simulink library "MIL_Test"  (Simulink 6.6)
undefined symbols (not defined in the file or in its folder): getdatatypespecs, slcm, StepSize
libraries: simulink x71, MIL_Test x6
(part 4 of 8)

== system MIL_Test/Validation Function/Feature extraction/Step response characteristics/Step response characteristics extraction/Extract steady state error ==
  Step response : Inport
  Set point : Inport  Port=2
  Subtract : Sum  Inputs=+-  OutScaling=2^-10
  Weighted Moving Average : S-Function  FunctionName=sfix_fir  Parameters=(getdatatypespecs(OutDataType,OutScaling,DblOver,0)),[DoSatur RndMeth-1],DblOver,dolog,mgainval,(getdatatypespecs(GainDataType,GainScaling,DblOver,RadixGroup)),samptime,vinit,OutputDataTypeScalingMode,GainDataTypeScalingMode  mask(Weighted Moving Average){mgainval=ones(1,10), vinit=0.0, samptime=-1, GainDataTypeScalingMode=Inherit via internal rule, GainDataType=sfix( 16 ), MatRadixGroup=Best Precision: Matrix-wise, GainScaling=2^-10, OutputDataTypeScalingMode=Inherit via internal rule, OutDataType=sfix(16), OutScaling=2^-10, LockScale=off, RndMeth=Floor, DoSatur=off}
      mask prompts: mgainval "Weights:"; vinit "Initial condition:"; samptime "Sample time:"; GainDataTypeScalingMode "Gain data type and scaling:"; GainDataType "Parameter data type:     ex. sfix(16),  uint(8), float('single')"; MatRadixGroup "Parameter scaling mode:"; GainScaling "Parameter scaling:    Slope    ex.  2^-9"; OutputDataTypeScalingMode "Output data type and scaling:"; OutDataType "Output data type:     ex.  sfix(16),  uint(8),  float('single')"; OutScaling "Output scaling:    Slope or [Slope Bias]    ex.  2^-9"; LockScale "Lock output scaling so autoscaling tool can't change it"; RndMeth "Round toward:"; DoSatur "Saturate to max or min when overflows occur"
      mask help: Output the weighted moving average of the input.
      mask init:
      | DblOver = 0;
      | dolog = 0;
      | 
      | if MatRadixGroup == 5
      |     RadixGroup = 1; % BEST_PREC_MAT
      | elseif MatRadixGroup == 4
      |     RadixGroup = 2; % BEST_PREC_COL
      | elseif MatRadixGroup == 3
      |     RadixGroup = 3; % BEST_PREC_ROW
      | elseif MatRadixGroup == 2
      |     RadixGroup = 4; % BEST_PREC_ELE
      | else
      |     RadixGroup = 0; % BEST_PREC_OFF
      | end
      mask StyleString: edit,edit,edit,popup(Specify via dialog|Inherit via internal rule),edit,popup(Use Specified Scaling|Best Precision: Element-wise|Best Precision: Row-wise|Best Precision: Column-wise|Best Precision: Matrix-wise),edit,popup(Specify via dialog|Inherit via internal rule|Inherit via back propagation),edit,edit,checkbox,popup(Zero|Nearest|Ceiling|Floor),checkbox
      mask CallbackString: |||fixptdialog(gcbh)|fixptdialog(gcbh)|fixptdialog(gcbh)||fixptdialog(gcbh)|fixptdialog(gcbh)||||
      mask TabNameString: Main,Main,Main,Parameter data types,Parameter data types,Parameter data types,Parameter data types,Signal data types,Signal data types,Signal data types,Signal data types,Signal data types,Signal data types
      mask Display:
      | fprintf(fixpt_fir_mask_data(mgainval,'dispstr'))
      | plot(fixpt_fir_mask_data(mgainval,1),fixpt_fir_mask_data(mgainval,0))
  ss error : Outport
  wires:
  Weighted Moving Average/1 -> ss error/1
  Subtract/1 -> Weighted Moving Average/1
  Set point/1 -> Subtract/2
  Step response/1 -> Subtract/1

== system MIL_Test/Validation Function/Feature extraction/Step response characteristics/Step response characteristics extraction/Step time ==
  Clock : Inport
  Trigger : TriggerPort
  Time : Outport
  wires:
  Clock/1 -> Time/1

== system MIL_Test/Validation Function/Feature extraction/Step response characteristics/Step response reset/Active if signals constant for some specified time ==
  Signal1 : Inport
  Signal 2 : Inport  Port=2
  Logical Operator1 : Logic  AllPortsSameDT=off  OutDataTypeMode=Boolean
  Min Time : Constant
  MinMax : MinMax  Inputs=2
  Relational Operator2 : RelationalOperator  Operator=<=  LogicOutDataTypeMode=Boolean
  Switch : Switch  Criteria=u2 ~= 0
  Time since signal constant : Subsystem  TreatAsAtomicUnit=on  mask(Feature extraction block){RT=0.0001}
      mask prompts: RT "Relative tolerance in %"
      mask help: Detect if the signal value is constant (using the last two signal values) allowing for a user-defined relative deviation
      mask CallbackString:
      | if or( (str2double(get_param(gcb,'RT')) < 0), (str2double(get_param(gcb,'RT')) > 100))
      |     error(['Relative tolerance value (' get_param(gcb,'RT') ') out of range. Please give a value between 0 and 100.']);
      | else
      |     set_param([gcb '/Detect constant/Relative tolerance/Relative Tolerance'],'Value',get_param(gcb,'RT'));
      |     set_param([gcb '/Detect constant'],'RT',get_param(gcb,'RT'));
      | end
  Time since signal constant1 : Subsystem  TreatAsAtomicUnit=on  mask(Feature extraction block){RT=0.0001}
      mask prompts: RT "Relative tolerance in %"
      mask help: Detect if the signal value is constant (using the last two signal values) allowing for a user-defined relative deviation
      mask CallbackString:
      | if or( (str2double(get_param(gcb,'RT')) < 0), (str2double(get_param(gcb,'RT')) > 100))
      |     error(['Relative tolerance value (' get_param(gcb,'RT') ') out of range. Please give a value between 0 and 100.']);
      | else
      |     set_param([gcb '/Detect constant/Relative tolerance/Relative Tolerance'],'Value',get_param(gcb,'RT'));
      |     set_param([gcb '/Detect constant'],'RT',get_param(gcb,'RT'));
      | end
  Zero : Constant  Value=0
  Constant signals : Outport
  wires:
  Zero/1 -> Switch/3
  Logical Operator1/1 -> Switch/2
  MinMax/1 -> Switch/1
  Time since signal constant1/1(Trigger) -> Logical Operator1/2
  Time since signal constant/1(Trigger) -> Logical Operator1/1
  Time since signal constant/2(Feature) -> MinMax/1
  Time since signal constant1/2(Feature) -> MinMax/2
  Switch/1 -> Relational Operator2/2
  Min Time/1 -> Relational Operator2/1
  Relational Operator2/1 -> Constant signals/1
  Signal 2/1 -> Time since signal constant1/1(Signal)
  Signal1/1 -> Time since signal constant/1(Signal)

== system MIL_Test/Validation Function/Feature extraction/Step response characteristics/Step response reset/Step detection ==
  Signal : Inport
  Abs : Abs
  Add : Sum  Inputs=+-  OutScaling=2^-10
  Clock : Clock
      settings: Decimation=10
  Memory : Memory
  Min step size : Constant
  Relational Operator : RelationalOperator  LogicOutDataTypeMode=Boolean
  Switch : Switch  Criteria=u2 > Threshold
  Step : Outport
  wires:
  Switch/1 -> Add/2
  Memory/1 -> Switch/1
  Clock/1 -> Switch/2
  Signal/1 -> Add/1, Switch/3, Memory/1
  Abs/1 -> Relational Operator/1
  Min step size/1 -> Relational Operator/2
  Relational Operator/1 -> Step/1
  Add/1 -> Abs/1

== system MIL_Test/Validation Function/Feature extraction/Step response characteristics/Step response trigger/Active if signals constant for some specified time ==
  Signal1 : Inport
  Signal 2 : Inport  Port=2
  Logical Operator1 : Logic  AllPortsSameDT=off  OutDataTypeMode=Boolean
  Min Time : Constant
  MinMax : MinMax  Inputs=2
  Relational Operator2 : RelationalOperator  Operator=<=  LogicOutDataTypeMode=Boolean
  Switch : Switch  Criteria=u2 ~= 0
  Time since signal constant : Subsystem  TreatAsAtomicUnit=on  mask(Feature extraction block){RT=0.5}
      mask prompts: RT "Relative tolerance in %"
      mask help: Detect if the signal value is constant (using the last two signal values) allowing for a user-defined relative deviation
      mask CallbackString:
      | if or( (str2double(get_param(gcb,'RT')) < 0), (str2double(get_param(gcb,'RT')) > 100))
      |     error(['Relative tolerance value (' get_param(gcb,'RT') ') out of range. Please give a value between 0 and 100.']);
      | else
      |     set_param([gcb '/Detect constant/Relative tolerance/Relative Tolerance'],'Value',get_param(gcb,'RT'));
      |     set_param([gcb '/Detect constant'],'RT',get_param(gcb,'RT'));
      | end
  Time since signal constant1 : Subsystem  TreatAsAtomicUnit=on  mask(Feature extraction block){RT=0.5}
      mask prompts: RT "Relative tolerance in %"
      mask help: Detect if the signal value is constant (using the last two signal values) allowing for a user-defined relative deviation
      mask CallbackString:
      | if or( (str2double(get_param(gcb,'RT')) < 0), (str2double(get_param(gcb,'RT')) > 100))
      |     error(['Relative tolerance value (' get_param(gcb,'RT') ') out of range. Please give a value between 0 and 100.']);
      | else
      |     set_param([gcb '/Detect constant/Relative tolerance/Relative Tolerance'],'Value',get_param(gcb,'RT'));
      |     set_param([gcb '/Detect constant'],'RT',get_param(gcb,'RT'));
      | end
  Zero : Constant  Value=0
  Constant signals : Outport
  wires:
  Zero/1 -> Switch/3
  Logical Operator1/1 -> Switch/2
  MinMax/1 -> Switch/1
  Time since signal constant1/1(Trigger) -> Logical Operator1/2
  Time since signal constant/1(Trigger) -> Logical Operator1/1
  Time since signal constant/2(Feature) -> MinMax/1
  Time since signal constant1/2(Feature) -> MinMax/2
  Switch/1 -> Relational Operator2/2
  Min Time/1 -> Relational Operator2/1
  Relational Operator2/1 -> Constant signals/1
  Signal 2/1 -> Time since signal constant1/1(Signal)
  Signal1/1 -> Time since signal constant/1(Signal)

== system MIL_Test/Validation Function/Feature extraction/Step response characteristics/Step response trigger/Compare To Constant ==
  u : Inport
  Compare : RelationalOperator  Operator=<=  LogicOutDataTypeMode=Specify via dialog  ZeroCross=off  InputSameDT=on
  Constant : Constant  Value=const  OutScaling=1
  y : Outport
  wires:
  u/1 -> Compare/1
  Constant/1 -> Compare/2
  Compare/1 -> y/1

== system MIL_Test/Validation Function/Feature extraction/Step response characteristics/Step response trigger/Detect increase ==
  Signal : Inport
  Clock : Clock
      settings: Decimation=10
  Memory : Memory
  Relational Operator : RelationalOperator  Operator=>  LogicOutDataTypeMode=Specify via dialog
  Switch : Switch  Criteria=u2 > Threshold
  Increase : Outport
  wires:
  Signal/1 -> Relational Operator/1, Memory/1, Switch/3
  Relational Operator/1 -> Increase/1
  Clock/1 -> Switch/2
  Memory/1 -> Switch/1
  Switch/1 -> Relational Operator/2

== system MIL_Test/Validation Function/Feature extraction/Time since signal constant/Detect constant/Relative tolerance ==
  sig : Inport
  ref : Inport  Port=2
  Abs : Abs
  Abs1 : Abs
  Add : Sum  Inputs=+-  OutScaling=2^-10
  Divide1 : Product  Inputs=**/  OutScaling=2^-10
  Max : Constant  Value=100
  Relational Operator : RelationalOperator  Operator=<=  LogicOutDataTypeMode=Boolean
  Relative Tolerance : Constant  Value=0.0001
  sig == ref : Outport
  wires:
  Abs1/1 -> Divide1/1
  Relational Operator/1 -> sig == ref/1
  Relative Tolerance/1 -> Divide1/2
  Max/1 -> Divide1/3
  Divide1/1 -> Relational Operator/2
  ref/1 -> Abs1/1, Add/2
  sig/1 -> Add/1
  Add/1 -> Abs/1
  Abs/1 -> Relational Operator/1

== system MIL_Test/Validation Function/TODO/<system name>/<Requirement name>/<Assertions name> ==
  Precond : Inport
  InOut Bus : Inport  Port=2
  <Reference name> : Constant
  Bus Creator : BusCreator  Inputs=1
  Bus Selector : BusSelector  OutputSignals=Inputs.signal1
  Feature extraction : Subsystem  TreatAsAtomicUnit=on  mask{Param=0}
      mask prompts: Param "Mask Parameter 1:"
  PAS : Subsystem  mask{AFT=TID, AFD=2}
      mask prompts: AFT "Assertion feature type:"; AFD "Assertion feature delay (in time steps)"
      mask init:
      | PAS_init(gcb);
      mask StyleString: popup(TI|TDD|TID),edit
      mask CallbackString: PAS_callback(gcb);|
  Signal comparison : Subsystem  TreatAsAtomicUnit=on  mask{Param=0}
      mask prompts: Param "Mask Parameter 1:"
  VF info : Outport
  wires:
  Bus Creator/1 -> VF info/1
  InOut Bus/1 -> Bus Selector/1
  Precond/1 -> PAS/1(Precond)
  PAS/1(VF Info) -> Bus Creator/1
  <Reference name>/1 -> Signal comparison/2(Ref)
  Feature extraction/3(A) -> Signal comparison/1(Sig)
  Feature extraction/2(T) -> PAS/3(T)
  Feature extraction/1(R) -> PAS/2(R)
  Bus Selector/1 -> Feature extraction/1(Sig)  "<signal1>"
  Signal comparison/1(V) -> PAS/4(V)

== system MIL_Test/Validation Function/TODO/<system name>/<Requirement name>/<Preconditions name> ==
  InOut Bus : Inport
  <Reference name> : Constant
  Bus Selector : BusSelector  OutputSignals=Inputs.signal1
  Feature extraction : Subsystem  TreatAsAtomicUnit=on  mask{Param=0}
      mask prompts: Param "Mask Parameter 1:"
  PS : Subsystem  mask(Feature layer: preconditions synchronization){NoTI=0, NoTDD=0, NoTID=1, TIdel=[0], TDDdel=[0]}
      mask prompts: NoTI "Time-independent features identifiable with or without a delay (TI)"; NoTDD "Triggered features identifiable with determinate delay or without a delay (TDD)"; NoTID "Triggered features identifiable with indeterminate delay (TID)"; TIdel "Time-independent features delays (in time steps). E.g. [0 1 0] for 3 features"; TDDdel "Triggered features delays (in time steps). E.g. [0 0] for 2 features"
      mask help: Use this block for synchronizing the precondition features. For changing the block inputs, use the parameters below. The output must be used for assertions activation.
      mask init:
      | PS_init(gcb);
      mask StyleString: popup(0|1|2|3|4|5|6|7|8|9),popup(0|1|2|3|4|5|6|7|8|9),popup(0|1|2|3|4|5|6|7|8|9),edit,edit
      mask CallbackString:
      | PSTI_callback(gcb);|PSTDD_callback(gcb);|PSTID_callback(gcb);|NoTI = str2double(get_param(gcb,'NoTI'));
      | TIdel = str2num(get_param(gcb,'TIdel'));
      | if NoTI ~= length(TIdel) && NoTI ~= 0
      |     error(['The number of delays entered (' num2str(length(TIdel)) ') does not correspond to the above specified number of time-independent features (' num2str(NoTI) ').']);
      | end|NoTDD = str2double(get_param(gcb,'NoTDD'));
      | TDDdel = str2num(get_param(gcb,'TDDdel'));
      | if NoTDD ~= length(TDDdel) && NoTDD ~= 0
      |     error(['The number of delays entered (' num2str(length(TDDdel)) ') does not correspond to the above specified number of triggered features with constant delay (' num2str(NoTDD) ').']);
      | end
  Signal comparison : Subsystem  TreatAsAtomicUnit=on  mask{Param=0}
      mask prompts: Param "Mask Parameter 1:"
  Activate : Outport
  wires:
  InOut Bus/1 -> Bus Selector/1
  PS/1(Precond) -> Activate/1
  Signal comparison/1(A) -> PS/3(A TID1)
  <Reference name>/1 -> Signal comparison/2(Ref)
  Feature extraction/3(A) -> Signal comparison/1(Sig)
  Feature extraction/2(T) -> PS/2(T TID1)
  Feature extraction/1(R) -> PS/1(R TID1)
  Bus Selector/1 -> Feature extraction/1(Sig)  "<signal1>"

== system MIL_Test/Validation Function/TODO/Assertions/Signal comparison/Bound ==
  Signal : Inport
  Reference : Inport  Port=2
  LOWER : Constant  Value=Lower  OutDataTypeMode=int8
  No Limit : Constant  Value=Inf
  No limit : Constant  Value=-Inf
  Relational Operator : RelationalOperator  LogicOutDataTypeMode=Specify via dialog
  Switch 1 : Switch  Criteria=u2 ~= 0
  Switch 2 : Switch  Criteria=u2 ~= 0
  UPPER : Constant  Value=Upper  OutDataTypeMode=int8
  Verdict : Outport
  Lower limit : Outport  Port=2
  Upper limit : Outport  Port=3
  wires:
  Switch 2/1 -> Upper limit/1
  Switch 1/1 -> Lower limit/1
  No limit/1 -> Switch 1/1
  LOWER/1 -> Switch 1/2
  No Limit/1 -> Switch 2/1
  UPPER/1 -> Switch 2/2
  Relational Operator/1 -> Verdict/1
  Signal/1 -> Relational Operator/1
  Reference/1 -> Switch 1/3, Switch 2/3, Relational Operator/2

== system MIL_Test/Validation Function/TODO/Assertions/Signal comparison/Range - Gap Absolute tolerance ==
  Signal : Inport
  Reference : Inport  Port=2
  Abs : Abs
  Absolute Tolerance : Constant  Value=AbsoluteTolerance
  Add : Sum  Inputs=+-  OutScaling=2^-10
  Add1 : Sum  Inputs=+-  OutScaling=2^-10
  Add2 : Sum  OutScaling=2^-10
  Relational Operator : RelationalOperator  Operator=<=  LogicOutDataTypeMode=Boolean
  Verdict : Outport
  LL : Outport  Port=2
  UL : Outport  Port=3
  wires:
  Absolute Tolerance/1 -> Add2/2, Add1/2, Relational Operator/2
  Reference/1 -> Add/2, Add1/1, Add2/1
  Signal/1 -> Add/1
  Add/1 -> Abs/1
  Abs/1 -> Relational Operator/1
  Relational Operator/1 -> Verdict/1
  Add1/1 -> LL/1
  Add2/1 -> UL/1

== system MIL_Test/Validation Function/TODO/Assertions/Signal comparison/Range - Gap Relative tolerance ==
  Signal : Inport
  Reference : Inport  Port=2
  Abs : Abs
  Add : Sum  Inputs=+-  OutScaling=2^-10
  Add1 : Sum  Inputs=+-  OutScaling=2^-10
  Add2 : Sum  OutScaling=2^-10
  Constant1 : Constant  Value=100
  Divide1 : Product  Inputs=**/  OutScaling=2^-10
  Relational Operator : RelationalOperator  Operator=<=  LogicOutDataTypeMode=Boolean
  Relative Tolerance : Constant  Value=RelativeTolerance
  Verdict : Outport
  LL : Outport  Port=2
  UL : Outport  Port=3
  wires:
  Add2/1 -> UL/1
  Add1/1 -> LL/1
  Relational Operator/1 -> Verdict/1
  Abs/1 -> Relational Operator/1
  Add/1 -> Abs/1
  Signal/1 -> Add/1
  Reference/1 -> Add2/1, Add1/1, Add/2, Divide1/1
  Divide1/1 -> Relational Operator/2, Add1/2, Add2/2
  Constant1/1 -> Divide1/3
  Relative Tolerance/1 -> Divide1/2

== system MIL_Test/Validation Function/TODO/Assertions/Signal comparison/Range - Gap Tolerance range ==
  Signal : Inport
  Lower bound : Inport  Port=2
  Upper bound : Inport  Port=3
  Logical Operator : Logic  AllPortsSameDT=off  OutDataTypeMode=Specify via dialog
  Relational Operator : RelationalOperator  LogicOutDataTypeMode=Boolean
  Relational Operator1 : RelationalOperator  LogicOutDataTypeMode=Boolean
  Verdict : Outport
  UL : Outport  Port=2
  LL : Outport  Port=3
  wires:
  Upper bound/1 -> Relational Operator1/1, UL/1
  Relational Operator/1 -> Logical Operator/2
  Relational Operator1/1 -> Logical Operator/1
  Signal/1 -> Relational Operator/1, Relational Operator1/2
  Logical Operator/1 -> Verdict/1
  Lower bound/1 -> LL/1, Relational Operator/2

== system MIL_Test/Validation Function/TODO/Preconditions/Signal comparison/Bound ==
  Signal : Inport
  Reference : Inport  Port=2
  RelOp : RelationalOperator  LogicOutDataTypeMode=Specify via dialog
  Verdict : Outport
  wires:
  Signal/1 -> RelOp/1
  RelOp/1 -> Verdict/1
  Reference/1 -> RelOp/2

== system MIL_Test/Validation Function/TODO/Preconditions/Signal comparison/Range - Gap Absolute tolerance ==
  Signal : Inport
  Reference : Inport  Port=2
  Abs : Abs
  Absolute Tolerance : Constant  Value=AbsoluteTolerance
  Add : Sum  Inputs=+-  OutScaling=2^-10
  Relational Operator : RelationalOperator  Operator=<=  LogicOutDataTypeMode=Boolean
  Verdict : Outport
  wires:
  Relational Operator/1 -> Verdict/1
  Abs/1 -> Relational Operator/1
  Add/1 -> Abs/1
  Signal/1 -> Add/1
  Reference/1 -> Add/2
  Absolute Tolerance/1 -> Relational Operator/2

== system MIL_Test/Validation Function/TODO/Preconditions/Signal comparison/Range - Gap Relative tolerance ==
  Signal : Inport
  Reference : Inport  Port=2
  Abs : Abs
  Add : Sum  Inputs=+-  OutScaling=2^-10
  Constant1 : Constant  Value=100
  Divide1 : Product  Inputs=**/  OutScaling=2^-10
  Relational Operator : RelationalOperator  Operator=<=  LogicOutDataTypeMode=Boolean
  Relative Tolerance : Constant  Value=RelativeTolerance
  Verdict : Outport
  wires:
  Relative Tolerance/1 -> Divide1/2
  Constant1/1 -> Divide1/3
  Divide1/1 -> Relational Operator/2
  Reference/1 -> Divide1/1, Add/2
  Signal/1 -> Add/1
  Add/1 -> Abs/1
  Abs/1 -> Relational Operator/1
  Relational Operator/1 -> Verdict/1

== system MIL_Test/Validation Function/TODO/Preconditions/Signal comparison/Range - Gap Tolerance range ==
  Signal : Inport
  Lower bound : Inport  Port=2
  Upper bound : Inport  Port=3
  Logical Operator : Logic  AllPortsSameDT=off  OutDataTypeMode=Specify via dialog
  Relational Operator : RelationalOperator  LogicOutDataTypeMode=Boolean
  Relational Operator1 : RelationalOperator  LogicOutDataTypeMode=Boolean
  Verdict : Outport
  wires:
  Lower bound/1 -> Relational Operator/2
  Logical Operator/1 -> Verdict/1
  Signal/1 -> Relational Operator1/2, Relational Operator/1
  Relational Operator1/1 -> Logical Operator/1
  Relational Operator/1 -> Logical Operator/2
  Upper bound/1 -> Relational Operator1/1

== system MIL_Test/Validation Function/TODO/Validation FunctionsTemplate/Requirement/Assertions ==
  Activate : Inport
  InOut Bus : Inport  Port=2
  Bus Selector : BusSelector  OutputSignals=Outputs.signal2.BrakePedal
  VF info : Outport
  wires:
  InOut Bus/1 -> Bus Selector/1

== system MIL_Test/Validation Function/TODO/Validation FunctionsTemplate/Requirement/Preconditions ==
  InOut Bus : Inport
  Bus Selector1 : BusSelector  OutputSignals=Inputs.signal2.phi_Brake
  Activate : Outport
  wires:
  InOut Bus/1 -> Bus Selector1/1

== system MIL_Test/Validation Function/TODO/Validation FunctionsTemplate/Requirement2/Assertions ==
  Activate : Inport
  InOut Bus : Inport  Port=2
  Bus Selector : BusSelector  OutputSignals=Outputs.signal2.BrakePedal
  VF info : Outport
  wires:
  InOut Bus/1 -> Bus Selector/1

== system MIL_Test/Validation Function/TODO/Validation FunctionsTemplate/Requirement2/Preconditions ==
  InOut Bus : Inport
  Bus Selector1 : BusSelector  OutputSignals=Inputs.signal2.phi_Brake
  Activate : Outport
  wires:
  InOut Bus/1 -> Bus Selector1/1

== system MIL_Test/Validation Function/Test Evaluation Architecture/<system name>/<Requirement name>/<Assertions name> ==
  Precond : Inport
  InOut Bus : Inport  Port=2
  <Reference name> : Constant
  Bus Creator : BusCreator  Inputs=1
  Bus Selector : BusSelector  OutputSignals=signal1
  Feature extraction : Subsystem  TreatAsAtomicUnit=on  mask{Param=0}
      mask prompts: Param "Mask Parameter 1:"
  PAS : Subsystem  mask{AFT=TID, AFD=600}
      mask prompts: AFT "Assertion feature type:"; AFD "Assertion feature delay (in time steps)"
      mask init:
      | PAS_init(gcb);
      mask StyleString: popup(TI|TDD|TID),edit
      mask CallbackString: PAS_callback(gcb);|
  Signal comparison : Subsystem  TreatAsAtomicUnit=on  mask{Param=0}
      mask prompts: Param "Mask Parameter 1:"
  VF info : Outport
  wires:
  Signal comparison/1(V) -> PAS/4(V)
  Bus Selector/1 -> Feature extraction/1(Sig)  "<signal1>"
  Feature extraction/1(R) -> PAS/2(R)
  Feature extraction/2(T) -> PAS/3(T)
  Feature extraction/3(A) -> Signal comparison/1(Sig)
  <Reference name>/1 -> Signal comparison/2(Ref)
  PAS/1(VF Info) -> Bus Creator/1
  Precond/1 -> PAS/1(Precond)
  InOut Bus/1 -> Bus Selector/1
  Bus Creator/1 -> VF info/1

== system MIL_Test/Validation Function/Test Evaluation Architecture/<system name>/<Requirement name>/<Preconditions name> ==
  InOut Bus : Inport
  <Reference name> : Constant
  Bus Selector : BusSelector  OutputSignals=signal1
  Feature extraction : Subsystem  TreatAsAtomicUnit=on  mask{Param=0}
      mask prompts: Param "Mask Parameter 1:"
  PS : Subsystem  mask(Feature layer: preconditions synchronization){NoTI=0, NoTDD=0, NoTID=1, TIdel=[0], TDDdel=[0]}
      mask prompts: NoTI "Time-independent features identifiable with or without a delay (TI)"; NoTDD "Triggered features identifiable with determinate delay or without a delay (TDD)"; NoTID "Triggered features identifiable with indeterminate delay (TID)"; TIdel "Time-independent features delays (in time steps). E.g. [0 1 0] for 3 features"; TDDdel "Triggered features delays (in time steps). E.g. [0 0] for 2 features"
      mask help: Use this block for synchronizing the precondition features. For changing the block inputs, use the parameters below. The output must be used for assertions activation.
      mask init:
      | PS_init(gcb);
      mask StyleString: popup(0|1|2|3|4|5|6|7|8|9),popup(0|1|2|3|4|5|6|7|8|9),popup(0|1|2|3|4|5|6|7|8|9),edit,edit
      mask CallbackString:
      | PSTI_callback(gcb);|PSTDD_callback(gcb);|PSTID_callback(gcb);|NoTI = str2double(get_param(gcb,'NoTI'));
      | TIdel = str2num(get_param(gcb,'TIdel'));
      | if NoTI ~= length(TIdel) && NoTI ~= 0
      |     error(['The number of delays entered (' num2str(length(TIdel)) ') does not correspond to the above specified number of time-independent features (' num2str(NoTI) ').']);
      | end|NoTDD = str2double(get_param(gcb,'NoTDD'));
      | TDDdel = str2num(get_param(gcb,'TDDdel'));
      | if NoTDD ~= length(TDDdel) && NoTDD ~= 0
      |     error(['The number of delays entered (' num2str(length(TDDdel)) ') does not correspond to the above specified number of triggered features with constant delay (' num2str(NoTDD) ').']);
      | end
  Signal comparison : Subsystem  TreatAsAtomicUnit=on  mask{Param=0}
      mask prompts: Param "Mask Parameter 1:"
  Activate : Outport
  wires:
  Bus Selector/1 -> Feature extraction/1(Sig)  "<signal1>"
  Feature extraction/1(R) -> PS/1(R TID1)
  Feature extraction/2(T) -> PS/2(T TID1)
  Feature extraction/3(A) -> Signal comparison/1(Sig)
  <Reference name>/1 -> Signal comparison/2(Ref)
  Signal comparison/1(A) -> PS/3(A TID1)
  PS/1(Precond) -> Activate/1
  InOut Bus/1 -> Bus Selector/1

== system MIL_Test/Test Control/Test Control Architecture/Connection Helpers/TestControl for  TestCases Sequencing NoMask/IF Signal@SimStopTime for TC = value1/if Signal@t for TC = pass ==
  @time : Inport
  Signal1 : Inport  Port=2
  ClockAtEnd : Clock
      settings: Decimation=10
  Relational Operator1 : RelationalOperator  LogicOutDataTypeMode=Boolean
  check in range : Subsystem  TreatAsAtomicUnit=on
  Control Seq1 : Outport
  wires:
  ClockAtEnd/1 -> Relational Operator1/1
  @time/1 -> Relational Operator1/2
  Signal1/1 -> check in range/2(Signal)
  check in range/1(Control Seq) -> Control Seq1/1
  Relational Operator1/1 -> check in range/1(@[time]), check in range/Enable

== system MIL_Test/Test Control/Test Control Architecture/Connection Helpers/TestControl for  TestCases Sequencing NoMask/IF Signal@SimStopTime for TC = value1/if false, then  TC4 for 200 ==
  Action Port : ActionPort
  Embedded MATLAB Function : Stateflow chart

== system MIL_Test/Test Control/Test Control Architecture/Connection Helpers/TestControl for  TestCases Sequencing NoMask/IF Signal@SimStopTime for TC = value1/if true, then  TC2 for 400 ==
  Action Port : ActionPort
  Embedded MATLAB Function : Stateflow chart

== system MIL_Test/Test Control/Test Control Architecture/Connection Helpers/TestControl for  TestCases Sequencing NoMask/IF signal @[timeUp, timeDown] for TC = value1/if Signal@ [TDown,TUp]  for TC = Value ==
  @timeDown : Inport
  @timeUp : Inport  Port=2
  Signal : Inport  Port=3
  ClockDuring : Clock
      settings: Decimation=10
  Logical Operator1 : Logic  AllPortsSameDT=off  OutDataTypeMode=Boolean
  Relational Operator1 : RelationalOperator  LogicOutDataTypeMode=Boolean
  Relational Operator2 : RelationalOperator  Operator=<=  LogicOutDataTypeMode=Boolean
  check in range : Subsystem  TreatAsAtomicUnit=on
  Control Seq : Outport
  wires:
  ClockDuring/1 -> Relational Operator1/1, Relational Operator2/1
  @timeDown/1 -> Relational Operator1/2
  @timeUp/1 -> Relational Operator2/2
  Relational Operator1/1 -> Logical Operator1/1
  Relational Operator2/1 -> Logical Operator1/2
  Logical Operator1/1 -> check in range/1(@[time]), check in range/Enable
  Signal/1 -> check in range/2(Signal)
  check in range/1(Control Seq) -> Control Seq/1

== system MIL_Test/Test Control/Test Control Architecture/Connection Helpers/TestControl for  TestCases Sequencing NoMask/IF signal@time for TC = value1/if Signal@t for TC = pass ==
  @time : Inport
  Signal1 : Inport  Port=2
  ClockAtTime : Clock
      settings: Decimation=10
  Relational Operator1 : RelationalOperator  LogicOutDataTypeMode=Boolean
  check in range : Subsystem  TreatAsAtomicUnit=on
  Control Seq : Outport
  wires:
  ClockAtTime/1 -> Relational Operator1/1
  @time/1 -> Relational Operator1/2
  Relational Operator1/1 -> check in range/1(@[time]), check in range/Enable
  Signal1/1 -> check in range/2(Signal)
  check in range/1(Control Seq) -> Control Seq/1

== system MIL_Test/Test Control/Test Control Architecture/Test Control Conditions/IF Signal@SimStopTime for TC = value1/if Signal@t for TC = pass/check in range ==
  @[time] : Inport
  Signal : Inport  Port=2
  Enable : EnablePort
  Logical Operator2 : Logic  AllPortsSameDT=off  OutDataTypeMode=Boolean
  Relational Operator : RelationalOperator  Operator===  LogicOutDataTypeMode=Boolean
  Value : Constant  Value=condition
  Control Seq : Outport  InitialOutput=[2]
  wires:
  @[time]/1 -> Logical Operator2/2
  Logical Operator2/1 -> Control Seq/1
  Relational Operator/1 -> Logical Operator2/1
  Value/1 -> Relational Operator/2
  Signal/1 -> Relational Operator/1

== system MIL_Test/Test Control/Test Control Architecture/Test Control Conditions/IF signal @[timeUp, timeDown] for TC = value1/if Signal@ [TDown,TUp]  for TC = Value/check in range ==
  @[time] : Inport
  Signal : Inport  Port=2
  Enable : EnablePort
  Logical Operator2 : Logic  AllPortsSameDT=off  OutDataTypeMode=Boolean
  Relational Operator : RelationalOperator  Operator===  LogicOutDataTypeMode=Boolean
  Value : Constant  Value=condition
  Control Seq : Outport  InitialOutput=[2]
  wires:
  @[time]/1 -> Logical Operator2/2
  Logical Operator2/1 -> Control Seq/1
  Relational Operator/1 -> Logical Operator2/1
  Value/1 -> Relational Operator/2
  Signal/1 -> Relational Operator/1

== system MIL_Test/Test Control/Test Control Architecture/Test Control Conditions/IF signal@time for TC = value1/if Signal@t for TC = pass/check in range ==
  @[time] : Inport
  Signal : Inport  Port=2
  Enable : EnablePort
  Logical Operator2 : Logic  AllPortsSameDT=off  OutDataTypeMode=Boolean
  Relational Operator : RelationalOperator  Operator===  LogicOutDataTypeMode=Boolean
  Value : Constant  Value=condition
  Control Seq : Outport  InitialOutput=[2]
  wires:
  @[time]/1 -> Logical Operator2/2
  Logical Operator2/1 -> Control Seq/1
  Relational Operator/1 -> Logical Operator2/1
  Value/1 -> Relational Operator/2
  Signal/1 -> Relational Operator/1

== system MIL_Test/Test Control/Test Control Architecture/Test Control Conditions/IF signal@time1/if Signal@t for TC = pass/check in range ==
  @[time] : Inport
  Signal : Inport  Port=2
  Enable : EnablePort
  Logical Operator2 : Logic  AllPortsSameDT=off  OutDataTypeMode=Boolean
  Relational Operator : RelationalOperator  Operator===  LogicOutDataTypeMode=Boolean
  Value : Constant  Value=condition
  Control Seq : Outport  InitialOutput=[2]
  wires:
  @[time]/1 -> Logical Operator2/2
  Logical Operator2/1 -> Control Seq/1
  Relational Operator/1 -> Logical Operator2/1
  Value/1 -> Relational Operator/2
  Signal/1 -> Relational Operator/1

== system MIL_Test/Test Data/Test Data Architecture/<Test data generator>/<Requirement name>/<Preconditions name>/<Check> ==
  Out Bus : Inport
  <Reference name> : Constant
  Bus Selector : BusSelector  OutputSignals=signal1
  Memory : Memory  X0=[1]
  Signal comparison : Subsystem  TreatAsAtomicUnit=on  mask{Param=0}
      mask prompts: Param "Mask Parameter 1:"
  A : Outport
  wires:
  Bus Selector/1 -> Memory/1  "<SUT output>"
  <Reference name>/1 -> Signal comparison/2(Ref)
  Memory/1 -> Signal comparison/1(Sig)
  Signal comparison/1(A) -> A/1
  Out Bus/1 -> Bus Selector/1

== system MIL_Test/Test Data/Test Data Architecture/<Test data generator>/<Requirement name>/<Preconditions name>/Feature generation ==
  <signal1> : Outport

== system MIL_Test/Test Data/Test Data Architecture/<Test data generator>/<Requirement name>/Initialisation & Stabilisation/<Feature generation> ==
  <signal1> : Outport

== system MIL_Test/Validation Function/Feature extraction/Complete step detection/Step detection/Active if signals constant for some specified time/Time since signal constant ==
  Signal : Inport
  Clock : Clock
      settings: Decimation=10
  Detect constant : Subsystem  TreatAsAtomicUnit=on  mask(Feature extraction block){RT=0.001}
      mask prompts: RT "Relative tolerance in %"
      mask help: Detect if the signal value is constant (using the last two signal values) allowing for a user-defined relative deviation
      mask CallbackString:
      | if or( (str2double(get_param(gcb,'RT')) < 0), (str2double(get_param(gcb,'RT')) > 100))
      |     error(['Relative tolerance value (' get_param(gcb,'RT') ') out of range. Please give a value between 0 and 100.']);
      | else
      |     set_param([gcb '/Relative tolerance/Relative Tolerance'],'Value',get_param(gcb,'RT'));
      | end
  Logical Operator : Logic  Operator=NAND  AllPortsSameDT=off  OutDataTypeMode=Boolean
  Logical Operator1 : Logic  Operator=NOT  AllPortsSameDT=off  OutDataTypeMode=Boolean
  Memory : Memory  Orientation=left
  Memory1 : Memory
  Subtract : Sum  Inputs=-+  OutScaling=2^-10
  Switch : Switch  Criteria=u2 > Threshold
  Trigger : Outport
  Feature : Outport  Port=2
  wires:
  Logical Operator/1 -> Switch/2
  Logical Operator1/1 -> Logical Operator/2
  Memory1/1 -> Logical Operator1/1
  Memory/1 -> Switch/1
  Switch/1 -> Memory/1, Subtract/1
  Clock/1 -> Switch/3, Subtract/2
  Subtract/1 -> Feature/1
  Detect constant/1(Constant) -> Memory1/1, Logical Operator/1, Trigger/1
  Signal/1 -> Detect constant/1(Signal)

== system MIL_Test/Validation Function/Feature extraction/Complete step detection/Step detection/Active if signals constant for some specified time/Time since signal constant1 ==
  Signal : Inport
  Clock : Clock
      settings: Decimation=10
  Detect constant : Subsystem  TreatAsAtomicUnit=on  mask(Feature extraction block){RT=0.001}
      mask prompts: RT "Relative tolerance in %"
      mask help: Detect if the signal value is constant (using the last two signal values) allowing for a user-defined relative deviation
      mask CallbackString:
      | if or( (str2double(get_param(gcb,'RT')) < 0), (str2double(get_param(gcb,'RT')) > 100))
      |     error(['Relative tolerance value (' get_param(gcb,'RT') ') out of range. Please give a value between 0 and 100.']);
      | else
      |     set_param([gcb '/Relative tolerance/Relative Tolerance'],'Value',get_param(gcb,'RT'));
      | end
  Logical Operator : Logic  Operator=NAND  AllPortsSameDT=off  OutDataTypeMode=Boolean
  Logical Operator1 : Logic  Operator=NOT  AllPortsSameDT=off  OutDataTypeMode=Boolean
  Memory : Memory  Orientation=left
  Memory1 : Memory
  Subtract : Sum  Inputs=-+  OutScaling=2^-10
  Switch : Switch  Criteria=u2 > Threshold
  Trigger : Outport
  Feature : Outport  Port=2
  wires:
  Signal/1 -> Detect constant/1(Signal)
  Detect constant/1(Constant) -> Trigger/1, Logical Operator/1, Memory1/1
  Subtract/1 -> Feature/1
  Clock/1 -> Subtract/2, Switch/3
  Switch/1 -> Subtract/1, Memory/1
  Memory/1 -> Switch/1
  Memory1/1 -> Logical Operator1/1
  Logical Operator1/1 -> Logical Operator/2
  Logical Operator/1 -> Switch/2

== system MIL_Test/Validation Function/Feature extraction/Complete step detection/Step detection/Detect constant/Relative tolerance ==
  sig : Inport
  ref : Inport  Port=2
  Abs : Abs
  Abs1 : Abs
  Add : Sum  Inputs=+-  OutScaling=2^-10
  Divide1 : Product  Inputs=**/  OutScaling=2^-10
  Max : Constant  Value=100
  Relational Operator : RelationalOperator  Operator=<=  LogicOutDataTypeMode=Boolean
  Relative Tolerance : Constant  Value=0.0001
  sig == ref : Outport
  wires:
  Abs/1 -> Relational Operator/1
  Add/1 -> Abs/1
  sig/1 -> Add/1
  ref/1 -> Add/2, Abs1/1
  Divide1/1 -> Relational Operator/2
  Max/1 -> Divide1/3
  Relative Tolerance/1 -> Divide1/2
  Relational Operator/1 -> sig == ref/1
  Abs1/1 -> Divide1/1

== system MIL_Test/Validation Function/Feature extraction/Complete step detection/Step detection reset/Active if signals constant for some specified time/Time since signal constant ==
  Signal : Inport
  Clock : Clock
      settings: Decimation=10
  Detect constant : Subsystem  TreatAsAtomicUnit=on  mask(Feature extraction block){RT=0.0001}
      mask prompts: RT "Relative tolerance in %"
      mask help: Detect if the signal value is constant (using the last two signal values) allowing for a user-defined relative deviation
      mask CallbackString:
      | if or( (str2double(get_param(gcb,'RT')) < 0), (str2double(get_param(gcb,'RT')) > 100))
      |     error(['Relative tolerance value (' get_param(gcb,'RT') ') out of range. Please give a value between 0 and 100.']);
      | else
      |     set_param([gcb '/Relative tolerance/Relative Tolerance'],'Value',get_param(gcb,'RT'));
      | end
  Logical Operator : Logic  Operator=NAND  AllPortsSameDT=off  OutDataTypeMode=Boolean
  Logical Operator1 : Logic  Operator=NOT  AllPortsSameDT=off  OutDataTypeMode=Boolean
  Memory : Memory  Orientation=left
  Memory1 : Memory
  Subtract : Sum  Inputs=-+  OutScaling=2^-10
  Switch : Switch  Criteria=u2 > Threshold
  Trigger : Outport
  Feature : Outport  Port=2
  wires:
  Logical Operator/1 -> Switch/2
  Logical Operator1/1 -> Logical Operator/2
  Memory1/1 -> Logical Operator1/1
  Memory/1 -> Switch/1
  Switch/1 -> Memory/1, Subtract/1
  Clock/1 -> Switch/3, Subtract/2
  Subtract/1 -> Feature/1
  Detect constant/1(Constant) -> Memory1/1, Logical Operator/1, Trigger/1
  Signal/1 -> Detect constant/1(Signal)

== system MIL_Test/Validation Function/Feature extraction/Complete step detection/Step detection reset/Active if signals constant for some specified time/Time since signal constant1 ==
  Signal : Inport
  Clock : Clock
      settings: Decimation=10
  Detect constant : Subsystem  TreatAsAtomicUnit=on  mask(Feature extraction block){RT=0.0001}
      mask prompts: RT "Relative tolerance in %"
      mask help: Detect if the signal value is constant (using the last two signal values) allowing for a user-defined relative deviation
      mask CallbackString:
      | if or( (str2double(get_param(gcb,'RT')) < 0), (str2double(get_param(gcb,'RT')) > 100))
      |     error(['Relative tolerance value (' get_param(gcb,'RT') ') out of range. Please give a value between 0 and 100.']);
      | else
      |     set_param([gcb '/Relative tolerance/Relative Tolerance'],'Value',get_param(gcb,'RT'));
      | end
  Logical Operator : Logic  Operator=NAND  AllPortsSameDT=off  OutDataTypeMode=Boolean
  Logical Operator1 : Logic  Operator=NOT  AllPortsSameDT=off  OutDataTypeMode=Boolean
  Memory : Memory  Orientation=left
  Memory1 : Memory
  Subtract : Sum  Inputs=-+  OutScaling=2^-10
  Switch : Switch  Criteria=u2 > Threshold
  Trigger : Outport
  Feature : Outport  Port=2
  wires:
  Signal/1 -> Detect constant/1(Signal)
  Detect constant/1(Constant) -> Trigger/1, Logical Operator/1, Memory1/1
  Subtract/1 -> Feature/1
  Clock/1 -> Subtract/2, Switch/3
  Switch/1 -> Subtract/1, Memory/1
  Memory/1 -> Switch/1
  Memory1/1 -> Logical Operator1/1
  Logical Operator1/1 -> Logical Operator/2
  Logical Operator/1 -> Switch/2

== system MIL_Test/Validation Function/Feature extraction/Step response characteristics/Step response characteristics extraction/Extract maximum overshoot/Active if signals constant for some specified time ==
  Signal1 : Inport
  Signal 2 : Inport  Port=2
  Logical Operator1 : Logic  AllPortsSameDT=off  OutDataTypeMode=Boolean
  Min Time : Constant  Value=0.1
  MinMax : MinMax  Inputs=2
  Relational Operator2 : RelationalOperator  Operator=<=  LogicOutDataTypeMode=Boolean
  Switch : Switch  Criteria=u2 ~= 0
  Time since signal constant : Subsystem  TreatAsAtomicUnit=on  mask(Feature extraction block){RT=0.1}
      mask prompts: RT "Relative tolerance in %"
      mask help: Detect if the signal value is constant (using the last two signal values) allowing for a user-defined relative deviation
      mask CallbackString:
      | if or( (str2double(get_param(gcb,'RT')) < 0), (str2double(get_param(gcb,'RT')) > 100))
      |     error(['Relative tolerance value (' get_param(gcb,'RT') ') out of range. Please give a value between 0 and 100.']);
      | else
      |     set_param([gcb '/Detect constant/Relative tolerance/Relative Tolerance'],'Value',get_param(gcb,'RT'));
      |     set_param([gcb '/Detect constant'],'RT',get_param(gcb,'RT'));
      | end
  Time since signal constant1 : Subsystem  TreatAsAtomicUnit=on  mask(Feature extraction block){RT=0.1}
      mask prompts: RT "Relative tolerance in %"
      mask help: Detect if the signal value is constant (using the last two signal values) allowing for a user-defined relative deviation
      mask CallbackString:
      | if or( (str2double(get_param(gcb,'RT')) < 0), (str2double(get_param(gcb,'RT')) > 100))
      |     error(['Relative tolerance value (' get_param(gcb,'RT') ') out of range. Please give a value between 0 and 100.']);
      | else
      |     set_param([gcb '/Detect constant/Relative tolerance/Relative Tolerance'],'Value',get_param(gcb,'RT'));
      |     set_param([gcb '/Detect constant'],'RT',get_param(gcb,'RT'));
      | end
  Zero : Constant  Value=0
  Constant signals : Outport
  wires:
  Zero/1 -> Switch/3
  Logical Operator1/1 -> Switch/2
  MinMax/1 -> Switch/1
  Time since signal constant1/1(Trigger) -> Logical Operator1/2
  Time since signal constant/1(Trigger) -> Logical Operator1/1
  Time since signal constant/2(Feature) -> MinMax/1
  Time since signal constant1/2(Feature) -> MinMax/2
  Switch/1 -> Relational Operator2/2
  Min Time/1 -> Relational Operator2/1
  Relational Operator2/1 -> Constant signals/1
  Signal 2/1 -> Time since signal constant1/1(Signal)
  Signal1/1 -> Time since signal constant/1(Signal)

== system MIL_Test/Validation Function/Feature extraction/Step response characteristics/Step response characteristics extraction/Extract maximum overshoot/Detect increase ==
  Signal : Inport
  Clock : Clock
      settings: Decimation=10
  Memory : Memory
  Relational Operator : RelationalOperator  Operator=>  LogicOutDataTypeMode=Specify via dialog
  Switch : Switch  Criteria=u2 > Threshold
  Increase : Outport
  wires:
  Signal/1 -> Relational Operator/1, Memory/1, Switch/3
  Relational Operator/1 -> Increase/1
  Clock/1 -> Switch/2
  Memory/1 -> Switch/1
  Switch/1 -> Relational Operator/2

== system MIL_Test/Validation Function/Feature extraction/Step response characteristics/Step response characteristics extraction/Extract maximum overshoot/Detect increase1 ==
  Signal : Inport
  Clock : Clock
      settings: Decimation=10
  Memory : Memory
  Relational Operator : RelationalOperator  Operator=>  LogicOutDataTypeMode=Specify via dialog
  Switch : Switch  Criteria=u2 > Threshold
  Increase : Outport
  wires:
  Signal/1 -> Relational Operator/1, Memory/1, Switch/3
  Relational Operator/1 -> Increase/1
  Clock/1 -> Switch/2
  Memory/1 -> Switch/1
  Switch/1 -> Relational Operator/2

== system MIL_Test/Validation Function/Feature extraction/Step response characteristics/Step response characteristics extraction/Extract maximum overshoot/Detect increase2 ==
  Signal : Inport
  Clock : Clock
      settings: Decimation=10
  Memory : Memory
  Relational Operator : RelationalOperator  Operator=>  LogicOutDataTypeMode=Specify via dialog
  Switch : Switch  Criteria=u2 > Threshold
  Increase : Outport
  wires:
  Switch/1 -> Relational Operator/2
  Memory/1 -> Switch/1
  Clock/1 -> Switch/2
  Relational Operator/1 -> Increase/1
  Signal/1 -> Switch/3, Memory/1, Relational Operator/1

== system MIL_Test/Validation Function/Feature extraction/Step response characteristics/Step response characteristics extraction/Extract maximum overshoot/Hold value with counter ==
  Reset counter : Inport
  Value : Inport  Port=2
  Trigger : TriggerPort
  Execution counter : Subsystem  TreatAsAtomicUnit=on
  Memory : Memory  InheritSampleTime=on
  Number of executions : Constant
  Relational Operator : RelationalOperator  Operator=<=  LogicOutDataTypeMode=Boolean
  Switch : Switch  Criteria=u2 ~= 0
  Held value : Outport
  wires:
  Relational Operator/1 -> Switch/2
  Execution counter/1(Counter) -> Relational Operator/1
  Number of executions/1 -> Relational Operator/2
  Reset counter/1 -> Execution counter/1(Reset)
  Value/1 -> Switch/1
  Switch/1 -> Held value/1, Memory/1
  Memory/1 -> Switch/3
